simulink model "B1P15_Torsonal_Model_With_RE_From_V_Rizzo_One_Coupler"  (Simulink 6.4)
settings: Solver=ode23tb  StartTime=0.0  StopTime=0.5  RelTol=1e-3
values from neighbouring files (symbols this model uses):
  Ka = 10    [B1P15_Torsonal_Model_From_V_Rizzo_One_Coupler_Constants.m]    (also in RizzoConst.m)
  Ke = 10    [B1P15_Torsonal_Model_From_V_Rizzo_One_Coupler_Constants.m]    (also in RizzoConst.m)
  Kr = 10    [B1P15_Torsonal_Model_From_V_Rizzo_One_Coupler_Constants.m]    (also in RizzoConst.m)
  Kt = 10    [B1P15_Torsonal_Model_From_V_Rizzo_One_Coupler_Constants.m]    (also in RizzoConst.m)
  Ms = 1/((Jm+JL)*s*F)    [B1P15_Torsonal_Model_From_V_Rizzo_One_Coupler_Constants.m]
  R = 10    [B1P15_Torsonal_Model_From_V_Rizzo_One_Coupler_Constants.m]    (also in RizzoConst.m)
undefined symbols (not defined in the file or in its folder): Hs, Ky, Y
settings Model: LastModifiedBy=Geovana

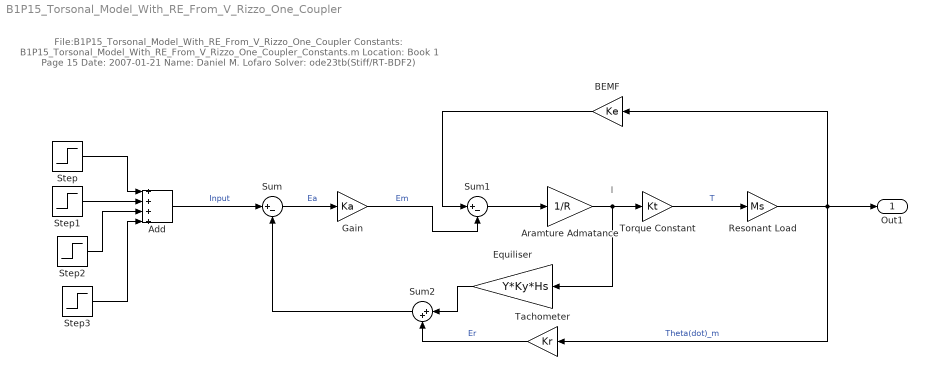
== system B1P15_Torsonal_Model_With_RE_From_V_Rizzo_One_Coupler ==
  note: File:B1P15_Torsonal_Model_With_RE_From_V_Rizzo_One_Coupler
      | Constants: B1P15_Torsonal_Model_With_RE_From_V_Rizzo_One_Coupler_Constants.m
      | Location: Book 1 Page 15
      | Date: 2007-01-21
      | Name: Daniel M. Lofaro
      | Solver: ode23tb(Stiff/RT-BDF2)
  note: I
  Add : Sum  Inputs=++++  OutScaling=2^-10
  Aramture Admatance : Gain  Gain=1/R
  BEMF : Gain  Orientation=left  Gain=Ke
  Equiliser : Gain  Orientation=left  Gain=Y*Ky*Hs
  Gain : Gain  Gain=Ka
  Resonant Load : Gain  Gain=Ms
  Step : Step  Time=0.1  SampleTime=0
  Step1 : Step  Time=0.2  After=-1  SampleTime=0
  Step2 : Step  Time=0.3  After=-1  SampleTime=0
  Step3 : Step  Time=0.4  SampleTime=0
  Sum : Sum  Inputs=|+-
  Sum1 : Sum  Inputs=|+-
  Sum2 : Sum  Orientation=left  Inputs=|++
  Tachometer : Gain  Orientation=left  Gain=Kr
  Torque Constant : Gain  Gain=Kt
  Out1 : Outport
  wires:
  Step/1 -> Add/1
  Step1/1 -> Add/2
  Step2/1 -> Add/3
  Step3/1 -> Add/4
  Add/1 -> Sum/1  "Input"
  Sum/1 -> Gain/1  "Ea"
  Sum1/1 -> Aramture Admatance/1
  Aramture Admatance/1 -> Torque Constant/1, Equiliser/1
  Torque Constant/1 -> Resonant Load/1  "T"
  BEMF/1 -> Sum1/1
  Gain/1 -> Sum1/2  "Em"
  Resonant Load/1 -> Out1/1, BEMF/1, Tachometer/1  "Theta(dot)_m"
  Tachometer/1 -> Sum2/2  "Er"
  Sum2/1 -> Sum/2
  Equiliser/1 -> Sum2/1
